simulink model "ACC_System_If__impl"  (R2017b)
settings: Solver=FixedStepDiscrete  StartTime=0.0  StopTime=10.0  FixedStep=1  RelTol=1e-3
PreLoadFcn:
  | sl_refresh_customizations
  | enum_Simulink
  | simulinkExportUnitCs
  | ACC_Parameters
  | ACCData
InitFcn:
  | checkUnitMismatch
model workspace (MAT data in the model file):
  ESD_URL = 'http://127.0.0.1:63320/node?ref=r%3Af6839c77-5b9d-441b-9a46-8668f7352d69%28A_ACC._50_ImplementationDefinitionHeterogeneous%29%2F1192123807590925316'
settings Model: Creator=eh6qym  LastModifiedBy=eh6qym
settings OptimizationCC: DefaultParameterBehavior=Inlined  PassReuseOutputArgsAs=Individual arguments  ZeroExternalMemoryAtStartup=off
settings DebuggingCC: SignalRangeChecking=error  InheritedTsInSrcMsg=none  ParameterTunabilityLossMsg=error
settings SFSimCC: MATLABDynamicMemAlloc=off
settings RTWCC: SystemTargetFile=esd_ert.tlc  GenCodeOnly=on  TemplateMakefile=ert_default_tmf  Description=CSD  GenerateReport=on  IncludeHyperlinkInReport=on  LaunchReport=on  GenerateTraceInfo=on  GenerateTraceReport=on  GenerateTraceReportSl=on  GenerateTraceReportSf=on  GenerateTraceReportEml=on
settings CodeAppCC: ForceParamTrailComments=on  IgnoreCustomStorageClasses=off  OperatorAnnotations=on  SimulinkDataObjDesc=on  SFDataObjDesc=on  InsertBlockDesc=on
settings STFCustomTargetCC: TargetLangStandard=C99 (ISO)  MultiwordLength=256  GenerateSampleERTMain=on  IncludeMdlTerminateFcn=off  CombineOutputUpdateFcns=on  CombineSignalStateStructs=on  SuppressErrorStatus=on  ERTCustomFileBanners=on  MultiInstanceERTCode=on  CodeInterfacePackaging=Reusable function  SupportContinuousTime=off  SupportNonInlinedSFcns=off  RemoveDisableFunc=on  RemoveResetFunc=on  MATLABClassNameForMDSCustomization=Simulink.SoftwareTarget.ERTCustomization  GRTInterface=off  SystemTargetFile=esd_ert.tlc
settings ERTTargetCC: TargetLangStandard=C99 (ISO)  GenerateSampleERTMain=on  ParMdlRefBuildCompliant=off  CompOptLevelCompliant=off  ConcurrentExecutionCompliant=off  IncludeMdlTerminateFcn=off  CombineSignalStateStructs=on  SuppressErrorStatus=on  MultiInstanceERTCode=on  CodeInterfacePackaging=Reusable function  RemoveDisableFunc=on  ModelStepFunctionPrototypeControlCompliant=off  CPPClassGenCompliant=off  UseToolchainInfoCompliant=off  InlinedParameterPlacement=NonHierarchical  ERTCustomFileTemplate=example_file_process.tlc

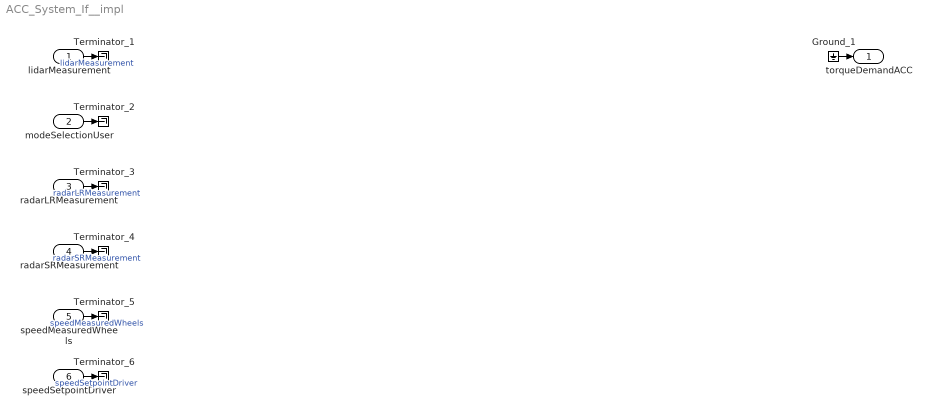
== system ACC_System_If__impl ==
  lidarMeasurement : Inport  OutDataTypeStr=double  Unit=m
      settings: AttributesFormatString=(m)
  modeSelectionUser : Inport  Port=2  OutDataTypeStr=Enum: ACCUserMode_t
  radarLRMeasurement : Inport  Port=3  OutDataTypeStr=double  Unit=m
      settings: AttributesFormatString=(m)
  radarSRMeasurement : Inport  Port=4  OutDataTypeStr=double  Unit=cm
      settings: AttributesFormatString=(cm)
  speedMeasuredWheels : Inport  Port=5  OutDataTypeStr=double  Unit=kmh
      settings: AttributesFormatString=(kmh)
  speedSetpointDriver : Inport  Port=6  OutDataTypeStr=double  Unit=kmh
      settings: AttributesFormatString=(kmh)
  Ground_1 : Ground
  Terminator_{1..6} (6 alike) : Terminator
  torqueDemandACC : Outport  OutDataTypeStr=double  Unit=Nm
      settings: AttributesFormatString=(Nm)
  wires:
  lidarMeasurement/1 -> Terminator_1/1  "lidarMeasurement"
  modeSelectionUser/1 -> Terminator_2/1
  radarLRMeasurement/1 -> Terminator_3/1  "radarLRMeasurement"
  radarSRMeasurement/1 -> Terminator_4/1  "radarSRMeasurement"
  speedMeasuredWheels/1 -> Terminator_5/1  "speedMeasuredWheels"
  speedSetpointDriver/1 -> Terminator_6/1  "speedSetpointDriver"
  Ground_1/1 -> torqueDemandACC/1
